simulink model "manipulatorTrajectoryFollow"  (R2022a)
settings: Solver=VariableStepAuto  StartTime=0.0  StopTime=5  MaxStep=0.1  RelTol=1e-2  AbsTol=1e-2
values from neighbouring files (symbols this model uses):
  dq0 = zeros(size(q0))    [manipulator_trajFollow_dataGen.m]
  jointLimits = jointLimits+jointLimitsTol.*repmat([-1,1],[size(jointLimits,1),1])    [manipulator_trajFollow_dataGen.m]
  q0 = traj(:,1)    [manipulator_trajFollow_dataGen.m]
  robot = loadrobot("rethinkSawyer","DataFormat","row")    [manipulator_RRT.m]    (also in manipulator_RRT_randomTrajs.m; manipulator_trajFollow_dataGen.m = importrobot('sawyer.urdf'))
  traj = path_set{i_traj,:}'    [manipulator_trajFollow_dataGen.m]
libraries: robotmaniplib x4, robotcorelib x1
settings Model: PauseTimes=3.1  Creator=The MathWorks, Inc.  LastModifiedBy=wulia
settings SolverCC: AlgebraicLoopSolver=TrustRegion
settings DebuggingCC: UnconnectedInputMsg=warning  UnconnectedOutputMsg=warning  UnconnectedLineMsg=warning  SFMachineParentedDataDiag=warning

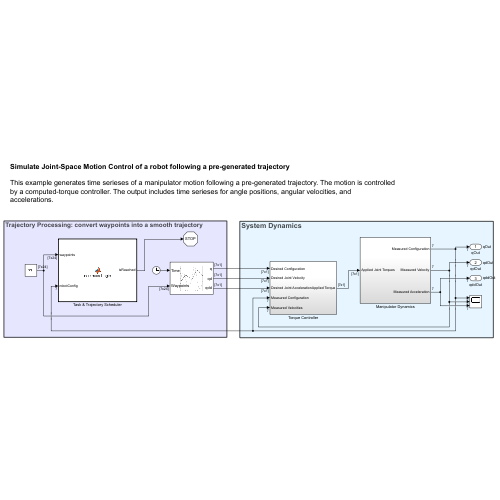
[thumbnail: Simulink's stored preview of the top-level diagram]
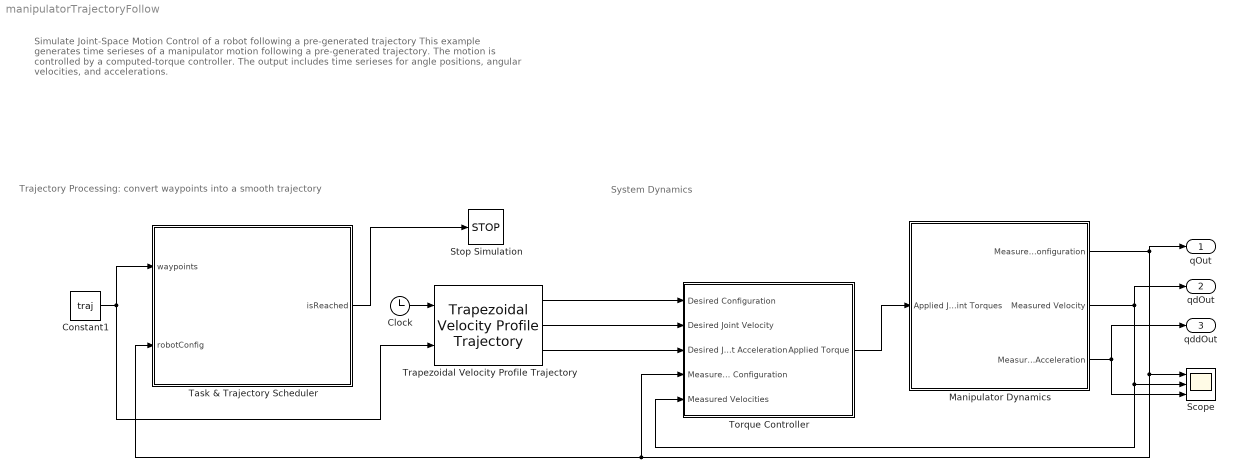
== system manipulatorTrajectoryFollow ==
  note: Trajectory Processing: convert waypoints into a smooth trajectory
  note: System Dynamics
  note: Simulate Joint-Space Motion Control of a robot following a pre-generated trajectory
      |
      | This example generates time serieses of a manipulator motion following a pre-generated trajectory. The motion is controlled by a computed-torque controller. The output includes time serieses for angle positions, angular velocities, and accelerations.
  Clock : Clock
  Constant1 : Constant  Value=traj  VectorParams1D=off
  Manipulator Dynamics : Subsystem
  Scope : Scope  NumInputPorts=3
  Stop Simulation : Stop
  Task & Trajectory Scheduler : MATLAB Function  TreatAsAtomicUnit=on
  Torque Controller : Subsystem
  Trapezoidal Velocity Profile Trajectory : robotcorelib/Trapezoidal Velocity Profile Trajectory  WaypointSource=External  Waypoints=[ 0, -0.5, -1; 0, 0.5, 1 ]  NumParams=1  Parameter1=End Time  Parameter2=Peak Velocity  ParameterSource=Internal  PeakVelocity=2*ones(7,1)  Acceleration=[ 1; 2 ]  EndTime=1  AccelTime=[ 1; 2 ]  SimulateUsing=Interpreted execution
      settings: SourceProductBaseCode=RO,NV,RR,UV
  qOut : Outport  SignalName=qOut
  qdOut : Outport  Port=2  SignalName=qdOut
  qddOut : Outport  Port=3  SignalName=qddOut
  wires:
  Constant1/1 -> Task & Trajectory Scheduler/1(waypoints), Trapezoidal Velocity Profile Trajectory/2
  Trapezoidal Velocity Profile Trajectory/1 -> Torque Controller/1(Desired Configuration)
  Trapezoidal Velocity Profile Trajectory/2 -> Torque Controller/2(Desired Joint Velocity)
  Trapezoidal Velocity Profile Trajectory/3 -> Torque Controller/3(Desired Joint Acceleration)
  Manipulator Dynamics/1(Measured Configuration) -> qOut/1, Task & Trajectory Scheduler/2(robotConfig), Torque Controller/4(Measured Configuration), Scope/1
  Manipulator Dynamics/2(Measured Velocity) -> qdOut/1, Scope/2, Torque Controller/5(Measured Velocities)
  Manipulator Dynamics/3(Measured Acceleration) -> qddOut/1, Scope/3
  Torque Controller/1(Applied Torque) -> Manipulator Dynamics/1(Applied Joint Torques)
  Clock/1 -> Trapezoidal Velocity Profile Trajectory/1
  Task & Trajectory Scheduler/1(isReached) -> Stop Simulation/1

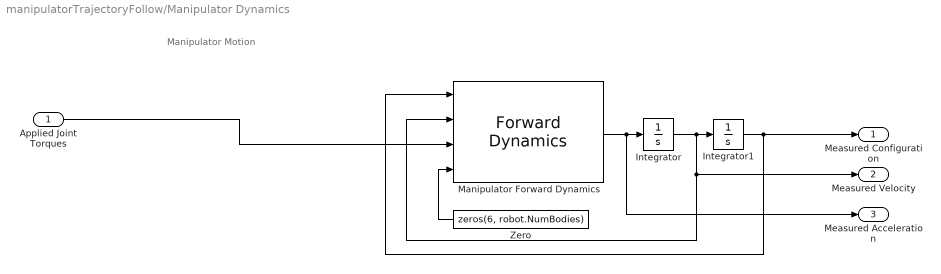
== system manipulatorTrajectoryFollow/Manipulator Dynamics ==
  note: Manipulator Motion
  Applied Joint Torques : Inport
  Integrator : Integrator  InitialCondition=dq0
  Integrator1 : Integrator  InitialCondition=q0  LimitOutput=on  UpperSaturationLimit=jointLimits(:,2)  LowerSaturationLimit=jointLimits(:,1)
  Manipulator Forward Dynamics : robotmaniplib/Forward Dynamics  RigidBodyTree=robot  SimulateUsing=Interpreted execution
  Zero : Constant  Value=zeros(6, robot.NumBodies)  OutDataTypeStr=Inherit: Inherit via back propagation
  Measured Configuration : Outport  VectorParamsAs1DForOutWhenUnconnected=off
  Measured Velocity : Outport  Port=2  VectorParamsAs1DForOutWhenUnconnected=off
  Measured Acceleration : Outport  Port=3  VectorParamsAs1DForOutWhenUnconnected=off
  wires:
  Zero/1 -> Manipulator Forward Dynamics/4
  Integrator/1 -> Manipulator Forward Dynamics/2, Measured Velocity/1, Integrator1/1
  Manipulator Forward Dynamics/1 -> Integrator/1, Measured Acceleration/1
  Applied Joint Torques/1 -> Manipulator Forward Dynamics/3
  Integrator1/1 -> Manipulator Forward Dynamics/1, Measured Configuration/1

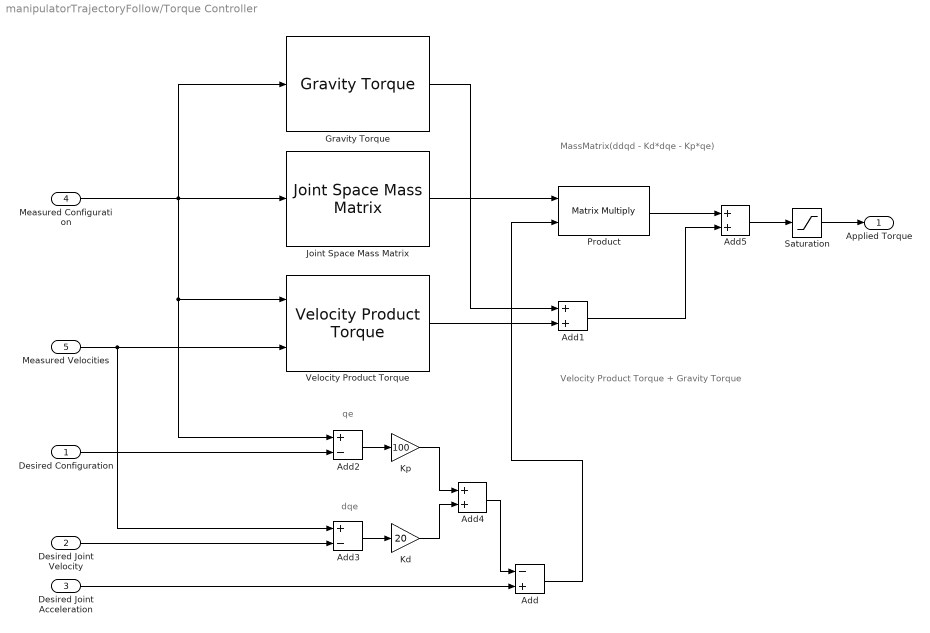
== system manipulatorTrajectoryFollow/Torque Controller ==
  note: MassMatrix(ddqd - Kd*dqe - Kp*qe)
  note: Velocity Product Torque + Gravity Torque
  note: dqe
  note: qe
  Desired Configuration : Inport
  Desired Joint Velocity : Inport  Port=2
  Desired Joint Acceleration : Inport  Port=3
  Measured Configuration : Inport  Port=4
  Measured Velocities : Inport  Port=5
  Add : Sum  Inputs=-+
  Add1 : Sum
  Add2 : Sum  Inputs=+-
  Add3 : Sum  Inputs=+-
  Add4 : Sum
  Add5 : Sum
  Gravity Torque : robotmaniplib/Gravity Torque  RigidBodyTree=robot  SimulateUsing=Interpreted execution
  Joint Space Mass Matrix : robotmaniplib/Joint Space Mass Matrix  RigidBodyTree=robot  SimulateUsing=Interpreted execution
  Kd : Gain  Gain=20
  Kp : Gain  Gain=100
  Product : Product  Multiplication=Matrix(*)
  Saturation : Saturate  UpperLimit=100  LowerLimit=-100
  Velocity Product Torque : robotmaniplib/Velocity Product Torque  RigidBodyTree=robot  SimulateUsing=Interpreted execution
      settings: SourceProductBaseCode=RO
  Applied Torque : Outport  VectorParamsAs1DForOutWhenUnconnected=off
  wires:
  Saturation/1 -> Applied Torque/1
  Velocity Product Torque/1 -> Add1/2
  Gravity Torque/1 -> Add1/1
  Add1/1 -> Add5/2
  Product/1 -> Add5/1
  Add5/1 -> Saturation/1
  Kd/1 -> Add4/2
  Kp/1 -> Add4/1
  Add3/1 -> Kd/1
  Add2/1 -> Kp/1
  Add/1 -> Product/2
  Add4/1 -> Add/1
  Measured Velocities/1 -> Velocity Product Torque/2, Add3/1
  Measured Configuration/1 -> Add2/1, Velocity Product Torque/1, Gravity Torque/1, Joint Space Mass Matrix/1
  Joint Space Mass Matrix/1 -> Product/1
  Desired Configuration/1 -> Add2/2
  Desired Joint Velocity/1 -> Add3/2
  Desired Joint Acceleration/1 -> Add/2

== matlab function manipulatorTrajectoryFollow/Task & Trajectory Scheduler ==
  settings: updateMethod=DISCRETE
  data: waypoints input; robotConfig input; isReached output
function isReached = commandLogic(waypoints, robotConfig)

% Set some variables
posTgtThreshold = 0.015;

% Initialize variables
isReached = false;

% Get the current status
trajEndConfigReached = endStateReached(robotConfig, waypoints, posTgtThreshold);

% Advance the state and reset time as needed
if trajEndConfigReached
    isReached = true;
end

end

function isReached = endStateReached(config, wpts, tgtThreshold)
    
    % Initialize output
    isReached = false;
    armTarget = wpts(:,end);
    
    % Check if the arm states match the target waypoints
    diffWpts = zeros(length(config),1);
    diffWpts(:,:) = abs(config - armTarget);
    errorStatus = diffWpts < tgtThreshold;
    if all(errorStatus)
        isReached = true;
    end
end
